simulink model "bilateral_teleoperation_PD"  (R2017a)
settings: Solver=FixedStepAuto  StartTime=0.0  StopTime=Inf  FixedStep=0.005  RelTol=1e-3  EnableMultiTasking=on
libraries: arduinolib x7, simulink x4
settings Model: SimulationMode=external  ExtModeTrigDuration=2  Creator=juanma  LastModifiedBy=juanma
settings OptimizationCC: PassReuseOutputArgsAs=Individual arguments  MaxStackSize=64
settings DebuggingCC: IntegerOverflowMsg=none  ParameterOverflowMsg=none  ParameterTunabilityLossMsg=error  IntegerSaturationMsg=none
settings HardwareCC: ProdBitPerInt=16  ProdBitPerPointer=16  ProdBitPerSizeT=16  ProdBitPerPtrDiffT=16  ProdLargestAtomicFloat=None  ProdWordSize=8  ProdHWDeviceType=Atmel->AVR
settings SFSimCC: MATLABDynamicMemAlloc=off
settings RTWCC: SystemTargetFile=ert.tlc  HardwareBoard=Arduino Mega 2560  TLCOptions=-aInlineSetEventsForThisBaseRateFcn=TLC_FALSE -aSuppressMultiTaskScheduler=TLC_FALSE -aRateBasedStepFcn=1  TemplateMakefile=ert_default_tmf  Description=Embedded Coder  GenerateReport=on  Toolchain=Arduino AVR  BuildConfiguration=Faster Runs  IncludeHyperlinkInReport=on  LaunchReport=on  GenerateTraceInfo=on  GenerateTraceReport=on  GenerateTraceReportSl=on  GenerateTraceReportSf=on  GenerateTraceReportEml=on
settings CodeAppCC: ForceParamTrailComments=on  IgnoreCustomStorageClasses=off  OperatorAnnotations=on  SimulinkDataObjDesc=on  SFDataObjDesc=on  MATLABFcnDesc=on  InsertBlockDesc=on  MATLABSourceComments=on
settings ERTTargetCC: SupportContinuousTime=on  SupportVariableSizeSignals=on

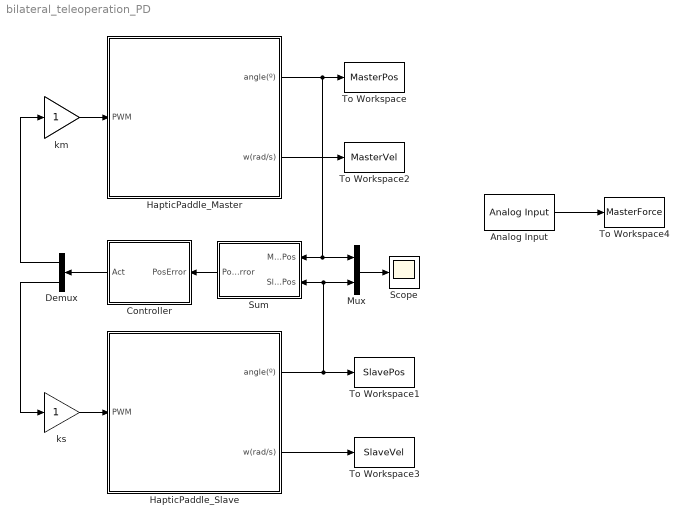
== system bilateral_teleoperation_PD ==
  Analog Input : arduinolib/Analog Input  pinNumber=8  sampleTime=-1  blockPlatform=arduino
  Controller : Subsystem
  Demux : Demux  Outputs=2
  HapticPaddle_Master : Subsystem
      mask Display:
      | pic=imread('haptic2017_render.png');
      | image(pic);
      | % color('blue');
      | % text(10, 10, 'HapticMega');
      | color('black');
      | port_label('Input', 1, 'PWM');
      | port_label('Output', 1, 'angle (º)');
      | port_label('Output', 2, 'w (rad/s)');
  HapticPaddle_Slave : Subsystem
      mask Display:
      | pic=imread('haptic2017_render.png');
      | image(pic);
      | % color('blue');
      | % text(10, 10, 'HapticMega');
      | color('black');
      | port_label('Input', 1, 'PWM');
      | port_label('Output', 1, 'angle (º)');
      | port_label('Output', 2, 'w (rad/s)');
  Mux : Mux  Inputs=2
  Scope : Scope
  Sum : Subsystem
  To Workspace : ToWorkspace  VariableName=MasterPos  SaveFormat=Structure With Time  SampleTime=-1
  To Workspace1 : ToWorkspace  VariableName=SlavePos  SaveFormat=Structure With Time  SampleTime=-1
  To Workspace2 : ToWorkspace  VariableName=MasterVel  SaveFormat=Structure With Time  SampleTime=-1
  To Workspace3 : ToWorkspace  VariableName=SlaveVel  SaveFormat=Structure With Time  SampleTime=-1
  To Workspace4 : ToWorkspace  VariableName=MasterForce  SaveFormat=Structure With Time  SampleTime=-1
  km : Gain  OutDataTypeStr=int16
  ks : Gain  OutDataTypeStr=int16
  wires:
  HapticPaddle_Slave/1(angle(º)) -> To Workspace1/1, Mux/2, Sum/2(SlavePos)
  HapticPaddle_Master/1(angle(º)) -> To Workspace/1, Mux/1, Sum/1(MasterPos)
  Mux/1 -> Scope/1
  HapticPaddle_Master/2(w(rad/s)) -> To Workspace2/1
  HapticPaddle_Slave/2(w(rad/s)) -> To Workspace3/1
  Sum/1(PosError) -> Controller/1(PosError)
  Controller/1(Act) -> Demux/1
  Demux/1 -> km/1
  Demux/2 -> ks/1
  ks/1 -> HapticPaddle_Slave/1(PWM)
  km/1 -> HapticPaddle_Master/1(PWM)
  Analog Input/1 -> To Workspace4/1

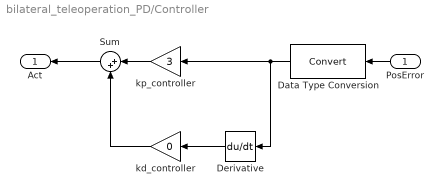
== system bilateral_teleoperation_PD/Controller ==
  PosError : Inport
  Data Type Conversion : DataTypeConversion
  Derivative : Derivative
  Sum : Sum  Inputs=|++
  kd_controller : Gain  Gain=0
  kp_controller : Gain  Gain=3
  Act : Outport
  wires:
  PosError/1 -> Data Type Conversion/1
  kp_controller/1 -> Sum/1
  Sum/1 -> Act/1
  Data Type Conversion/1 -> kp_controller/1, Derivative/1
  Derivative/1 -> kd_controller/1
  kd_controller/1 -> Sum/2

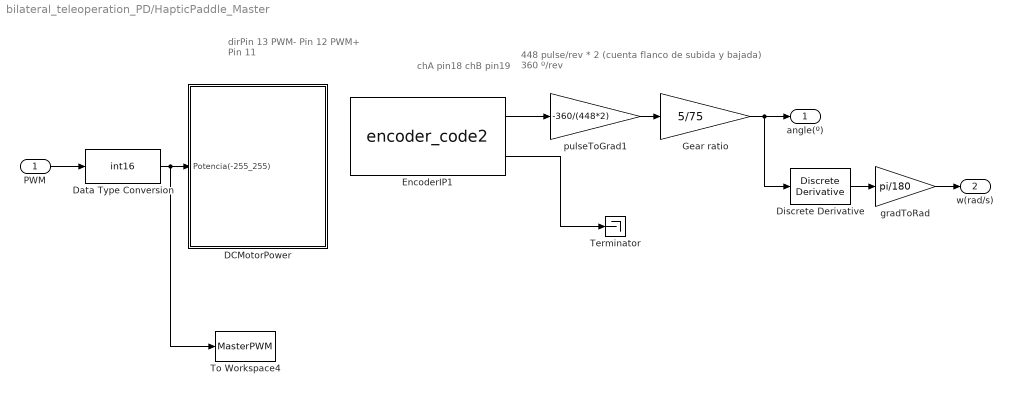
== system bilateral_teleoperation_PD/HapticPaddle_Master ==
  note: dirPin 13
      | PWM- Pin 12
      | PWM+ Pin 11
  note: chA pin18
      | chB pin19
  note: 448 pulse/rev * 2 (cuenta flanco de subida y bajada)
      | 360 º/rev
  PWM : Inport
  DCMotorPower : Subsystem
      settings: RTWFcnNameOpts=Use subsystem name  RTWFileNameOpts=Use function name
      mask Display:
      | pic=imread('L298.jpg');
      | image(pic,[0.28 0.18 0.45 0.65]);
      | 
      | color('blue');
      | text(0.1, 0.87, 'Puente H', 'horizontalAlignment', 'left');
      | color('black');
      | port_label('Input', 1, 'PWM');
  Data Type Conversion : DataTypeConversion  OutDataTypeStr=int16
  Discrete Derivative : simulink/Discrete/Discrete Derivative  gainval=1  ICPrevScaledInput=0.0  InputProcessing=Inherited  OutMin=[]  OutMax=[]  OutDataTypeStr=double  OutputDataTypeScalingMode=double  OutDataType=fixdt(1, 16)  OutScaling=2^-10  DoSatur=off
  EncoderIP1 : S-Function  InitFcn=try, set_param(gcb,'FunctionName','encoder_code2'), end  FunctionName=encoder_code2  Parameters=uint8(1),uint8(18),uint8(19)  SFunctionModules=encoder_code2_wrapper  SFunctionDeploymentMode=off  EnableBusSupport=off  mask(S-Function Builder){}
      mask init:
      | val = [[.9  0.75 0.75 1 1 .9 .9 1]',[1 1 0.75 0.75 .9 .9 1 .9]'];try , sys = get_param(gcb,'SfunBuilderFcnName');if isempty(sys), sys = get_param(gcb,'FunctionName'); end,catch, sys = get_param(gcb,'FunctionName'); end
      settings: CopyFcn=set_param(gcbh,'LinkStatus','none')  PreSaveFcn=try, set_param(gcb,'FunctionName','encoder_code2'), end  OpenFcn=sfunctionwizard(gcbh)
      mask Display: plot(val(:,1),val(:,2)),disp(sys), port_label('output',1,'pos'), port_label('output',2,'time')
  "Gear ratio " : Gain  Gain=5/75
  Terminator : Terminator
  To Workspace4 : ToWorkspace  VariableName=MasterPWM  SaveFormat=Structure With Time  SampleTime=-1
  gradToRad : Gain  Gain=pi/180
  pulseToGrad1 : Gain  Gain=-360/(448*2)
  angle(º) : Outport
  w(rad/s) : Outport  Port=2
  wires:
  gradToRad/1 -> w(rad/s)/1
  Discrete Derivative/1 -> gradToRad/1
  PWM/1 -> Data Type Conversion/1
  pulseToGrad1/1 -> "Gear ratio "/1
  "Gear ratio "/1 -> Discrete Derivative/1, angle(º)/1
  Data Type Conversion/1 -> To Workspace4/1, DCMotorPower/1("Potencia(-255_255) ")
  EncoderIP1/1 -> pulseToGrad1/1
  EncoderIP1/2 -> Terminator/1

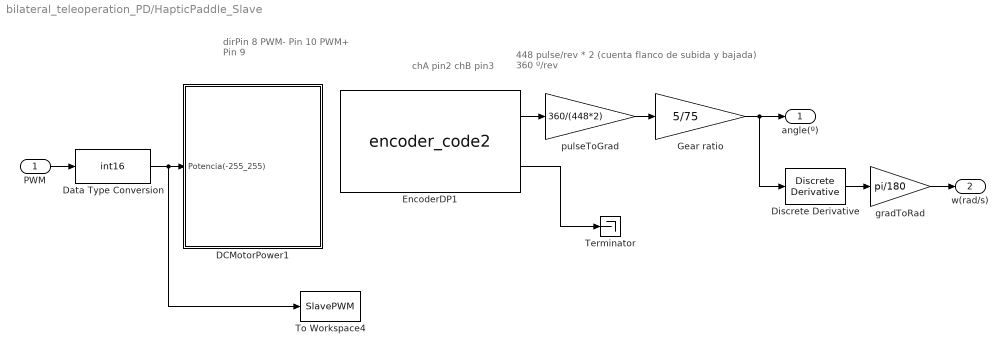
== system bilateral_teleoperation_PD/HapticPaddle_Slave ==
  note: dirPin 8
      | PWM- Pin 10
      | PWM+ Pin 9
  note: chA pin2
      | chB pin3
  note: 448 pulse/rev * 2 (cuenta flanco de subida y bajada)
      | 360 º/rev
  PWM : Inport
  DCMotorPower1 : Subsystem
      settings: RTWFcnNameOpts=Use subsystem name  RTWFileNameOpts=Use function name
      mask Display:
      | pic=imread('L298.jpg');
      | image(pic,[0.28 0.18 0.45 0.65]);
      | 
      | color('blue');
      | text(0.1, 0.87, 'Puente H', 'horizontalAlignment', 'left');
      | color('black');
      | port_label('Input', 1, 'PWM');
  Data Type Conversion : DataTypeConversion  OutDataTypeStr=int16
  Discrete Derivative : simulink/Discrete/Discrete Derivative  gainval=1  ICPrevScaledInput=0.0  InputProcessing=Inherited  OutMin=[]  OutMax=[]  OutDataTypeStr=double  OutputDataTypeScalingMode=double  OutDataType=fixdt(1, 16)  OutScaling=2^-10  DoSatur=off
  EncoderDP1 : S-Function  InitFcn=try, set_param(gcb,'FunctionName','encoder_code2'), end  FunctionName=encoder_code2  Parameters=uint8(0),uint8(2),uint8(3)  SFunctionModules=encoder_code2_wrapper  SFunctionDeploymentMode=off  EnableBusSupport=off  mask(S-Function Builder){}
      mask init: same as bilateral_teleoperation_PD/HapticPaddle_Master/EncoderIP1
      settings: CopyFcn=set_param(gcbh,'LinkStatus','none')  PreSaveFcn=try, set_param(gcb,'FunctionName','encoder_code2'), end  OpenFcn=sfunctionwizard(gcbh)
      mask Display: plot(val(:,1),val(:,2)),disp(sys), port_label('output',1,'pos'), port_label('output',2,'time')
  "Gear ratio " : Gain  Gain=5/75
  Terminator : Terminator
  To Workspace4 : ToWorkspace  VariableName=SlavePWM  SaveFormat=Structure With Time  SampleTime=-1
  gradToRad : Gain  Gain=pi/180
  pulseToGrad : Gain  Gain=360/(448*2)
  angle(º) : Outport
  w(rad/s) : Outport  Port=2
  wires:
  gradToRad/1 -> w(rad/s)/1
  Discrete Derivative/1 -> gradToRad/1
  PWM/1 -> Data Type Conversion/1
  pulseToGrad/1 -> "Gear ratio "/1
  "Gear ratio "/1 -> Discrete Derivative/1, angle(º)/1
  Data Type Conversion/1 -> To Workspace4/1, DCMotorPower1/1("Potencia(-255_255) ")
  EncoderDP1/2 -> Terminator/1
  EncoderDP1/1 -> pulseToGrad/1

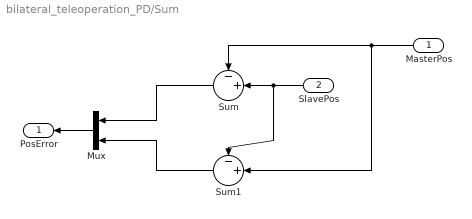
== system bilateral_teleoperation_PD/Sum ==
  MasterPos : Inport
  SlavePos : Inport  Port=2
  Mux : Mux  Inputs=2
  Sum : Sum  Inputs=-+|
  Sum1 : Sum  Inputs=-+|
  PosError : Outport
  wires:
  MasterPos/1 -> Sum1/2, Sum/1
  SlavePos/1 -> Sum1/1, Sum/2
  Sum/1 -> Mux/1
  Mux/1 -> PosError/1
  Sum1/1 -> Mux/2

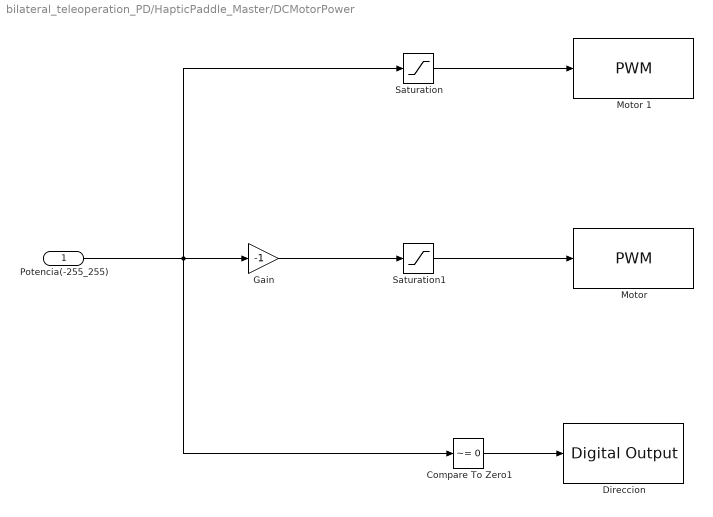
== system bilateral_teleoperation_PD/HapticPaddle_Master/DCMotorPower ==
  "Potencia(-255_255) " : Inport  OutDataTypeStr=int16
  Compare To Zero1 : simulink/Logic and Bit Operations/Compare To Zero  relop=~=  OutDataTypeStr=boolean
  Direccion : arduinolib/Digital Output  pinNumber=13  blockPlatform=arduino
  Gain : Gain  Gain=-1
  Motor : arduinolib/PWM  pinNumber=11  blockPlatform=arduino
  Motor 1 : arduinolib/PWM  pinNumber=12  blockPlatform=arduino
  Saturation : Saturate  UpperLimit=255  LowerLimit=0
  Saturation1 : Saturate  UpperLimit=255  LowerLimit=0
  wires:
  Saturation/1 -> Motor 1/1
  Compare To Zero1/1 -> Direccion/1
  Saturation1/1 -> Motor/1
  Gain/1 -> Saturation1/1
  "Potencia(-255_255) "/1 -> Saturation/1, Compare To Zero1/1, Gain/1

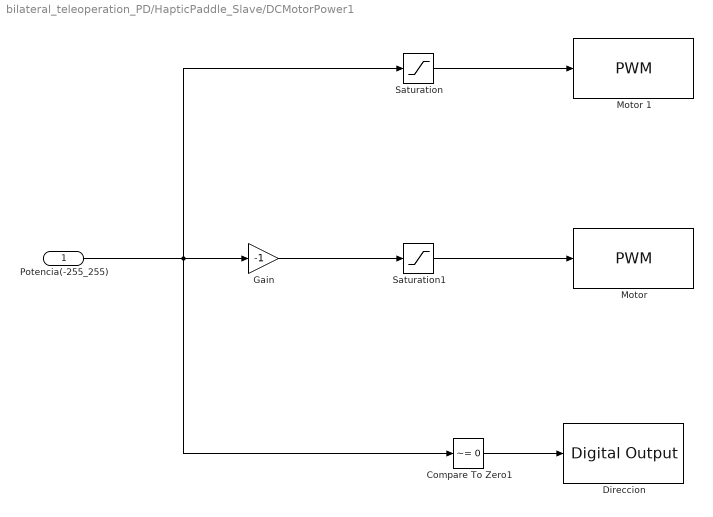
== system bilateral_teleoperation_PD/HapticPaddle_Slave/DCMotorPower1 ==
  "Potencia(-255_255) " : Inport  OutDataTypeStr=int16
  Compare To Zero1 : simulink/Logic and Bit Operations/Compare To Zero  relop=~=  OutDataTypeStr=boolean
  Direccion : arduinolib/Digital Output  pinNumber=8  blockPlatform=arduino
  Gain : Gain  Gain=-1
  Motor : arduinolib/PWM  pinNumber=10  blockPlatform=arduino
  Motor 1 : arduinolib/PWM  pinNumber=9  blockPlatform=arduino
  Saturation : Saturate  UpperLimit=255  LowerLimit=0
  Saturation1 : Saturate  UpperLimit=255  LowerLimit=0
  wires:
  Saturation/1 -> Motor 1/1
  Compare To Zero1/1 -> Direccion/1
  Saturation1/1 -> Motor/1
  Gain/1 -> Saturation1/1
  "Potencia(-255_255) "/1 -> Saturation/1, Compare To Zero1/1, Gain/1
